simulink model "flowchart_implementation"  (R2020a)
settings: Solver=VariableStepAuto  StartTime=0.0  StopTime=10.0  RelTol=1e-3
settings Model: Creator=Ganesh  LastModifiedBy=Ganesh

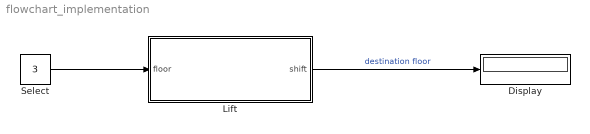
== system flowchart_implementation ==
  Display : Display
  Lift : Stateflow chart  TreatAsAtomicUnit=on
  Select : Constant  Value=3
  wires:
  Select/1 -> Lift/1(floor)
  Lift/1(shift) -> Display/1  "destination floor"

== stateflow chart flowchart_implementation/Lift ==
  (default) -> (junction 3) : {current =0;shift=0;}
  (junction 14) -> (junction 3) [order 1] : [current~=floor]
  (junction 3) -> (junction 5) [order 1] : [current<=floor && floor<6]
  (junction 3) -> (junction 6) [order 2]
  (junction 5) -> (junction 16) : {current=current+1;}
  (junction 6) -> (junction 12) [order 1] : [current>=floor && floor<6]
  (junction 6) -> (junction 14) [order 2] : {current=0;}
  (junction 12) -> (junction 15) : {current = current -1;}
  (junction 15) -> (junction 14)
  (junction 16) -> (junction 15)
  (junction 14) -> (junction 17) [order 2] : {shift =current;}
  data: floor input; shift output; current local =0
